simulink model "Plant"  (R2020a)
settings: Solver=VariableStepAuto  StartTime=0.0  StopTime=100  RelTol=1e-3
PreLoadFcn:
  | m = 1000;
  | b = 50;
  | u = 500;
settings Model: DataDictionary=Dictionary_Problem3.sldd  Creator=Admin  LastModifiedBy=Admin
settings DataIOCC: SaveOutput=off  SaveTime=off

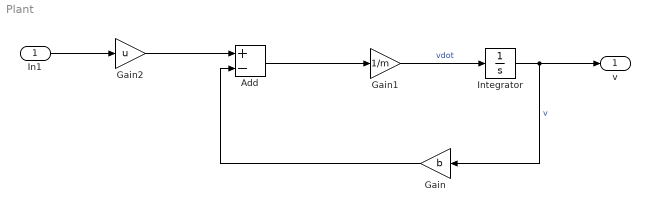
== system Plant ==
  In1 : Inport  OutDataTypeStr=double  PortDimensions=1  SampleTime=0
  Add : Sum  Inputs=+-
  Gain : Gain  Gain=b
  Gain1 : Gain  Gain=1/m
  Gain2 : Gain  Gain=u
  Integrator : Integrator
  v : Outport  OutDataTypeStr=double  PortDimensions=1  SampleTime=0
  wires:
  Gain2/1 -> Add/1
  Integrator/1 -> Gain/1, v/1  "v"
  Gain/1 -> Add/2
  Add/1 -> Gain1/1
  Gain1/1 -> Integrator/1  "vdot"
  In1/1 -> Gain2/1
